simulink model "trash"  (R2021a)
settings: Solver=VariableStepAuto  StartTime=0.0  StopTime=10.0  RelTol=1e-3
libraries: hdlsllib x6, simulink x2
settings Model: Creator=sbetu  LastModifiedBy=sbetu

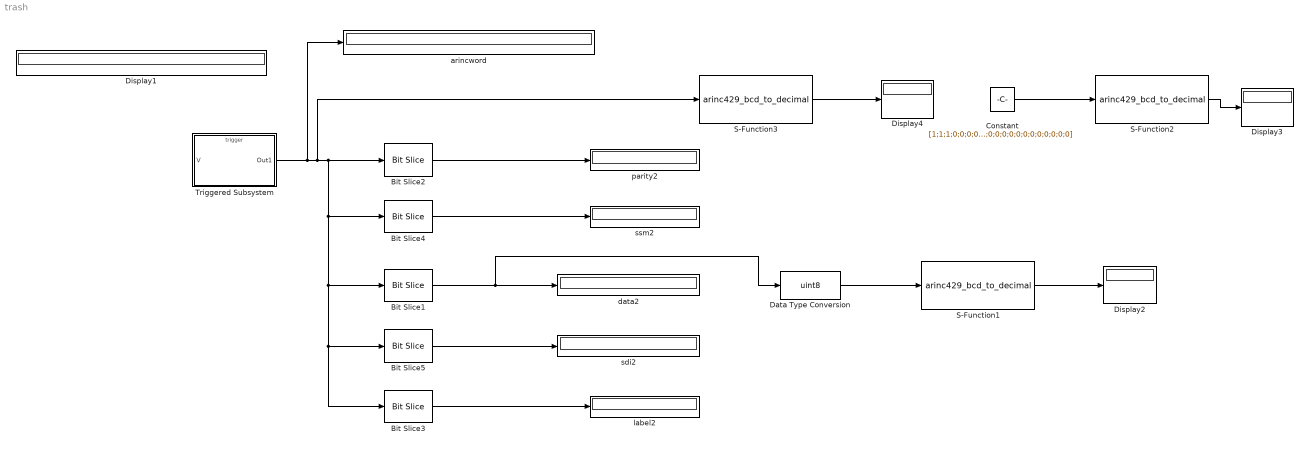
== system trash ==
  Bit Slice1 : hdlsllib/Logic and Bit Operations/Bit Slice  lidx=29  ridx=11
      settings: SourceProductBaseCode=SL
  Bit Slice2 : hdlsllib/Logic and Bit Operations/Bit Slice  lidx=32  ridx=32
      settings: SourceProductBaseCode=SL
  Bit Slice3 : hdlsllib/Logic and Bit Operations/Bit Slice  lidx=8  ridx=1
      settings: SourceProductBaseCode=SL
  Bit Slice4 : hdlsllib/Logic and Bit Operations/Bit Slice  lidx=31  ridx=30
      settings: SourceProductBaseCode=SL
  Bit Slice5 : hdlsllib/Logic and Bit Operations/Bit Slice  lidx=10  ridx=9
      settings: SourceProductBaseCode=SL
  Constant : Constant  Value=[1;1;1;0;0;0;0;0;0;0;0;0;0;0;0;0;0;0;0]  OutDataTypeStr=uint8
  Data Type Conversion : DataTypeConversion  OutDataTypeStr=uint8
  Display{1..4} (4 alike) : Display
      Display1 settings: Format=binary (Stored Integer)
  S-Function1 : S-Function  FunctionName=arinc429_bcd_to_decimal  SFunctionDeploymentMode=off  EnableBusSupport=off
  S-Function2 : S-Function  FunctionName=arinc429_bcd_to_decimal  SFunctionDeploymentMode=off  EnableBusSupport=off
  S-Function3 : S-Function  FunctionName=arinc429_bcd_to_decimal  SFunctionDeploymentMode=off  EnableBusSupport=off
  Triggered Subsystem : Subsystem  TreatAsAtomicUnit=on
  arincword : Display
      settings: Format=binary (Stored Integer)
  data2 : Display
      settings: Format=binary (Stored Integer)
  label2 : Display
      settings: Format=binary (Stored Integer)
  parity2 : Display
      settings: Format=binary (Stored Integer)
  sdi2 : Display
      settings: Format=binary (Stored Integer)
  ssm2 : Display
      settings: Format=binary (Stored Integer)
  wires:
  S-Function3/1 -> Display4/1
  Bit Slice1/1 -> Data Type Conversion/1, data2/1
  Bit Slice3/1 -> label2/1
  Constant/1 -> S-Function2/1
  S-Function1/1 -> Display2/1
  Bit Slice5/1 -> sdi2/1
  Triggered Subsystem/1(Out1) -> arincword/1, S-Function3/1, Bit Slice2/1, Bit Slice5/1, Bit Slice3/1, Bit Slice1/1, Bit Slice4/1
  ? -> Triggered Subsystem/Trigger  "clock"
  Data Type Conversion/1 -> S-Function1/1
  Bit Slice4/1 -> ssm2/1
  S-Function2/1 -> Display3/1
  Bit Slice2/1 -> parity2/1
  ? -> Display1/1, Triggered Subsystem/1(V)

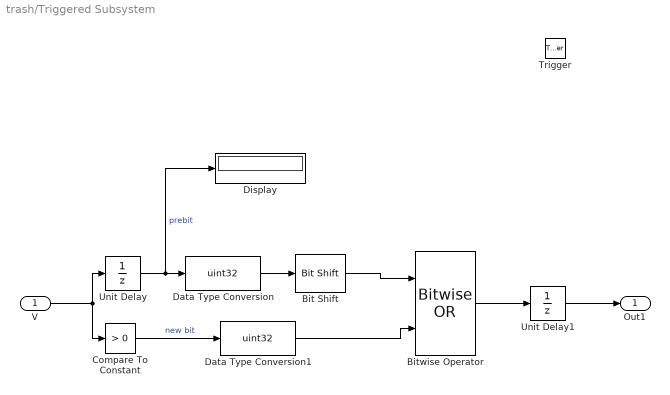
== system trash/Triggered Subsystem ==
  V : Inport
  Trigger : TriggerPort  VariantControl=(inherit)
  Bit Shift : hdlsllib/Logic and Bit Operations/Bit Shift  mode=Shift Left Logical  N=1
  Bitwise Operator : simulink/Logic and Bit Operations/Bitwise Operator  logicop=OR  UseBitMask=off  NumInputPorts=2  BitMask=bin2dec('11011001')  BitMaskRealWorld=Stored Integer
  Compare To Constant : simulink/Logic and Bit Operations/Compare To Constant  relop=>  const=0  OutDataTypeStr=boolean
  Data Type Conversion : DataTypeConversion  OutDataTypeStr=uint32
  Data Type Conversion1 : DataTypeConversion  OutDataTypeStr=uint32
  Display : Display
  Unit Delay : UnitDelay  SampleTime=-1  HasFrameUpgradeWarning=on
  Unit Delay1 : UnitDelay  SampleTime=-1  HasFrameUpgradeWarning=on
  Out1 : Outport
  wires:
  V/1 -> Unit Delay/1, Compare To Constant/1
  Unit Delay/1 -> Display/1, Data Type Conversion/1  "prebit"
  Bitwise Operator/1 -> Unit Delay1/1
  Unit Delay1/1 -> Out1/1
  Compare To Constant/1 -> Data Type Conversion1/1  "new bit"
  Bit Shift/1 -> Bitwise Operator/1
  Data Type Conversion/1 -> Bit Shift/1
  Data Type Conversion1/1 -> Bitwise Operator/2
